simulink model ""  (R2025a)
settings: Solver=VariableStepAuto  StartTime=0.0  StopTime=10.0  RelTol=1e-3
settings Model: ExtModeTrigDuration=100  Creator=adam  LastModifiedBy=adam

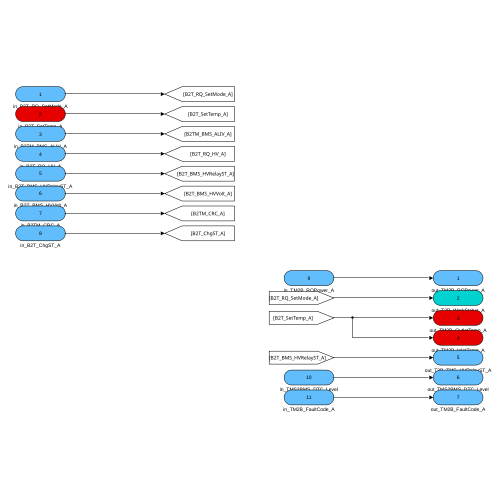
[thumbnail: Simulink's stored preview of the top-level diagram]
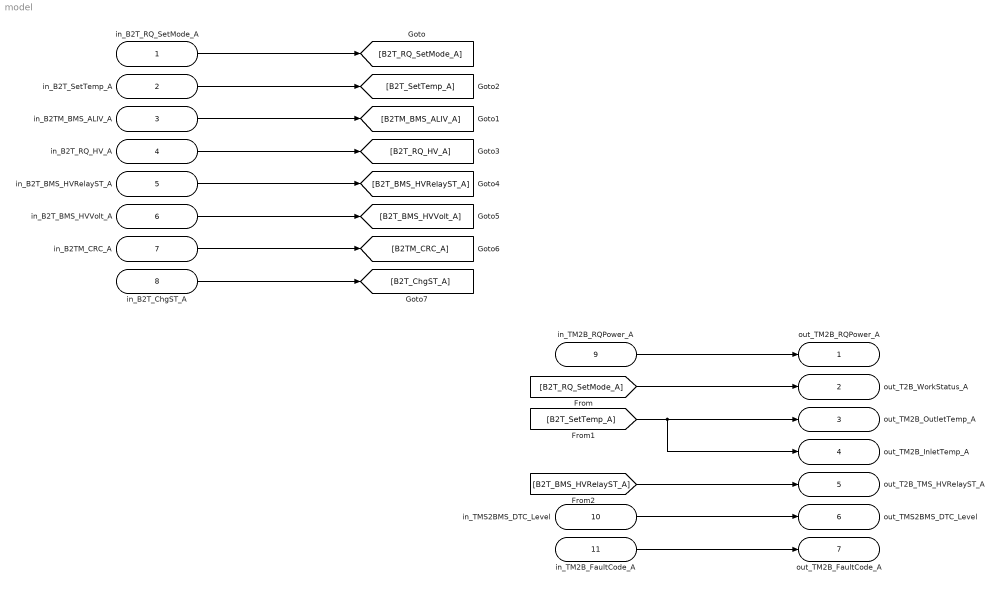
== system model ==
  in_B2T_RQ_SetMode_A : Inport
  in_B2T_SetTemp_A : Inport  Port=2
  in_B2TM_BMS_ALIV_A : Inport  Port=3
  in_B2T_RQ_HV_A : Inport  Port=4
  in_B2T_BMS_HVRelayST_A : Inport  Port=5
  in_B2T_BMS_HVVolt_A : Inport  Port=6
  in_B2TM_CRC_A : Inport  Port=7
  in_B2T_ChgST_A : Inport  Port=8
  in_TM2B_RQPower_A : Inport  Port=9
  in_TMS2BMS_DTC_Level : Inport  Port=10
  in_TM2B_FaultCode_A : Inport  Port=11
  out_TM2B_RQPower_A : Outport
  out_T2B_WorkStatus_A : Outport  Port=2
  out_TM2B_OutletTemp_A : Outport  Port=3
  out_TM2B_InletTemp_A : Outport  Port=4
  out_T2B_TMS_HVRelayST_A : Outport  Port=5
  out_TMS2BMS_DTC_Level : Outport  Port=6
  out_TM2B_FaultCode_A : Outport  Port=7
  wires:
  in_B2T_BMS_HVRelayST_A/1 -> [B2T_BMS_HVRelayST_A]
  in_B2T_RQ_HV_A/1 -> [B2T_RQ_HV_A]
  in_B2T_ChgST_A/1 -> [B2T_ChgST_A]
  in_B2TM_BMS_ALIV_A/1 -> [B2TM_BMS_ALIV_A]
  in_B2T_BMS_HVVolt_A/1 -> [B2T_BMS_HVVolt_A]
  in_B2T_SetTemp_A/1 -> [B2T_SetTemp_A]
  in_B2T_RQ_SetMode_A/1 -> [B2T_RQ_SetMode_A]
  in_B2TM_CRC_A/1 -> [B2TM_CRC_A]
  in_TM2B_RQPower_A/1 -> out_TM2B_RQPower_A/1
  [B2T_RQ_SetMode_A] -> out_T2B_WorkStatus_A/1
  [B2T_BMS_HVRelayST_A] -> out_T2B_TMS_HVRelayST_A/1
  in_TMS2BMS_DTC_Level/1 -> out_TMS2BMS_DTC_Level/1
  in_TM2B_FaultCode_A/1 -> out_TM2B_FaultCode_A/1
  [B2T_SetTemp_A] -> out_TM2B_InletTemp_A/1, out_TM2B_OutletTemp_A/1
